simulink model "odqsim_lft"  (R2016b)
settings: Solver=FixedStepDiscrete  StartTime=0.0  StopTime=10.0  FixedStep=Ts  RelTol=1e-3
values from neighbouring files (symbols this model uses):
  G = odqdata.G    [odqlab_interact.m]    (also in odqlab_verify.m; odqsim.m = varargin{1})
  Q = odqanly(G)    [odq.m]    (also in odqlab_interact.m = odqdata.Q; odqlab_verify.m = odqdata.Q; odqreal.m = orderfields(Q); odqsim.m = varargin{2})
undefined symbols (not defined in the file or in its folder): Ts
libraries: odqblock x3
settings Model: Creator=morita  LastModifiedBy=morita

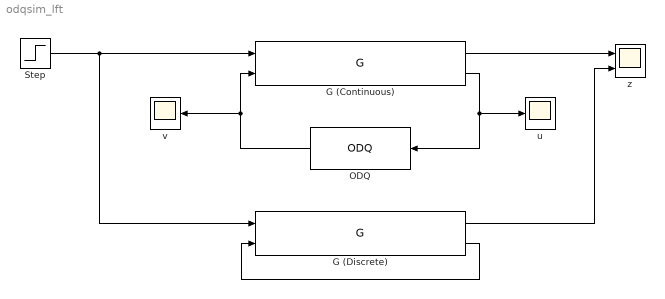
== system odqsim_lft ==
  G (Continuous) : odqblock/G  A=G.a  B1=G.b1  B2=G.b2  C1=G.c1  C2=G.c2  D1=G.d1  D2=G.d2  Ts=Ts  x0=x0
  G (Discrete) : odqblock/G  A=G.a  B1=G.b1  B2=G.b2  C1=G.c1  C2=G.c2  D1=G.d1  D2=G.d2  Ts=Ts  x0=x0
  ODQ : odqblock/ODQ  A=Q.a  B1=Q.b1  B2=Q.b2  C=Q.c  d=d  Ts=Ts
  Step : Step  Time=0  SampleTime=0
  u : Scope
  v : Scope
  z : Scope  NumInputPorts=2
  wires:
  G (Discrete)/1 -> z/2
  Step/1 -> G (Discrete)/1, G (Continuous)/1
  G (Continuous)/1 -> z/1
  G (Discrete)/2 -> G (Discrete)/2
  G (Continuous)/2 -> u/1, ODQ/1
  ODQ/1 -> v/1, G (Continuous)/2
